simulink model "nlsysid"  (Simulink 4.00)
settings: Solver=ode45  StartTime=0.0  StopTime=U(end,1)  RelTol=1e-3
values from neighbouring files (symbols this model uses):
  b = .5    (= 0.5)    [linid.m]    (also in nonlinid.m)
  h = 0.1    [linid.m]    (also in nonlinid.m = 0.05)
  x0 = [2;0]    [linid.m]    (also in nonlinid.m = [0;0])
settings Model: LastModifiedBy=R.Babuska

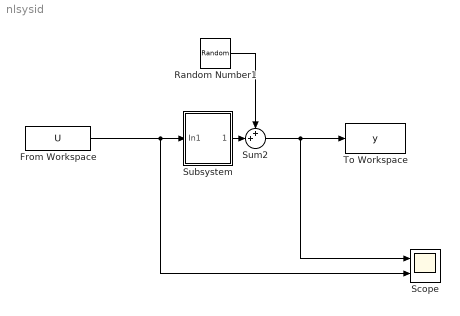
== system nlsysid ==
  From Workspace : FromWorkspace  VariableName=U  SampleTime=h  OutputAfterFinalValue=Extrapolation
  Random Number1 : RandomNumber  Mean=0  Variance=1e-5  Seed=0  SampleTime=h
  Scope : Scope  NumInputPorts=2
      settings: TimeRange=50  YMin=1.6~7  YMax=2.4~9  SaveToWorkspace=off  SaveName=ScopeData  LimitDataPoints=on  MaxDataPoints=5000  SampleInput=on  SampleTime=h
  Subsystem : Subsystem
      settings: RTWFcnNameOpts=Auto  RTWFileNameOpts=Auto
  Sum2 : Sum  Inputs=++|  SaturateOnIntegerOverflow=on
  To Workspace : ToWorkspace  VariableName=y  SampleTime=h  SaveFormat=Array
  wires:
  From Workspace/1 -> Subsystem/1(In1), Scope/2
  Sum2/1 -> Scope/1, To Workspace/1
  Subsystem/1(Out1) -> Sum2/2
  Random Number1/1 -> Sum2/1

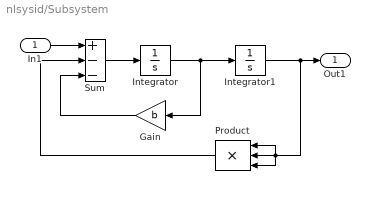
== system nlsysid/Subsystem ==
  In1 : Inport  Port=1  LatchInput=off
  Gain : Gain  Orientation=left  Gain=b  Multiplication=Element-wise(K.*u)  SaturateOnIntegerOverflow=on
  Integrator : Integrator  ExternalReset=none  InitialConditionSource=internal  InitialCondition=x0(2)  LimitOutput=off  UpperSaturationLimit=inf  LowerSaturationLimit=-inf  ShowSaturationPort=off  ShowStatePort=off  AbsoluteTolerance=auto
  Integrator1 : Integrator  ExternalReset=none  InitialConditionSource=internal  InitialCondition=x0(1)  LimitOutput=off  UpperSaturationLimit=inf  LowerSaturationLimit=-inf  ShowSaturationPort=off  ShowStatePort=off  AbsoluteTolerance=auto
  Product : Product  Orientation=left  Inputs=3  Multiplication=Element-wise(.*)  SaturateOnIntegerOverflow=on
  Sum : Sum  Inputs=+--  SaturateOnIntegerOverflow=on
  Out1 : Outport  Port=1
  wires:
  Integrator/1 -> Integrator1/1, Gain/1
  Sum/1 -> Integrator/1
  Integrator1/1 -> Product/2, Product/1, Product/3, Out1/1
  Product/1 -> Sum/2
  Gain/1 -> Sum/3
  In1/1 -> Sum/1
